simulink model "gtm_aeromodel"  (Simulink 7.2)
settings: Solver=ode45  StartTime=0.0  StopTime=10.0  RelTol=1e-3
undefined symbols (not defined in the file or in its folder): A_BLCG, A_BW, A_CW, A_FSCG, A_FSREF_in, A_SW, A_WLCG, A_WLREF, ALPHA0, bclowb, bclowbx_FMACH, bcmowb, bcmowbx_FHP, bcmowby_FMACH, cda, cdax_FLPDEF, cddr, cddrx_FMACH, cdo, cdox_FLPDEF, cdt1, cdt1x_mach, cdt2, cdt2x_mach, cdto, cdtox_mach, cdwb, cdwbx_FALPHA, cdwby_FMACH, clat, clatfr, clatfrx_FHP, clatfry_FMACH, clatx_mach, clawbfr, clawbfrx_FHP, clawbfry_FMACH, cldefr, cldefrx_FHP, cldefry_FMACH, cldtab, cldtabx_FMACH, clqwb, clqwbfr, clqwbfrx_FHP, clqwbfry_FMACH, clqwbx_mach, cltdd, cltddx_FHP, cltddy_FMACH, clwb, clwbtdd, clwbtddx_FHP, clwbtddy_FMACH, clwbx_FALPHA, clwby_FMACH, clwbzdd, clwbzddx_FHP, clwbzddy_FMACH, clzdd ... (+196)
libraries: model_lib x1
(part 8 of 10)

== system gtm_aeromodel/get aero forces and moments/AERODYNAMICS/Force  Coefficients/LIFT/CLWB/CLWBFLEX ==
  note: tddco2g=fqadot*fcbar/(2*32.174)
  altitude : Inport  OutDataType=sfix(16)  OutScaling=2^0
  Mach : Inport  Port=2  OutDataType=sfix(16)  OutScaling=2^0
  norm acc g's : Inport  Port=3  OutDataType=sfix(16)  OutScaling=2^0
  qdot : Inport  Port=4  OutDataType=sfix(16)  OutScaling=2^0
  Enable : EnablePort
  Fcn1 : Fcn  Expr=1/u
  Product1 : Product  OutDataType=sfix(16)  OutScaling=2^0  SaturateOnIntegerOverflow=on  RndMeth=Zero  InputSameDT=on  OutDataTypeStr=Inherit: Same as first input
  Product2 : Product  Inputs=3  OutDataType=sfix(16)  OutScaling=2^0  SaturateOnIntegerOverflow=on  RndMeth=Zero  InputSameDT=on  OutDataTypeStr=Inherit: Same as first input
  Product3 : Product  OutDataType=sfix(16)  OutScaling=2^0  SaturateOnIntegerOverflow=on  RndMeth=Zero  InputSameDT=on  OutDataTypeStr=Inherit: Same as first input
  Product4 : Product  OutDataType=sfix(16)  OutScaling=2^0  SaturateOnIntegerOverflow=on  RndMeth=Zero  InputSameDT=on  OutDataTypeStr=Inherit: Same as first input
  Sum3 : Sum  OutDataType=sfix(16)  OutScaling=2^0  SaturateOnIntegerOverflow=on  InputSameDT=on  OutDataTypeStr=Inherit: Same as first input
  Wing Chord : Constant  Value=A_CW  OutDataType=sfix(16)  OutScaling=2^0
  Wing Chord1 : Constant  Value=2  OutDataType=sfix(16)  OutScaling=2^0
  Wing Chord2 : Constant  Value=constants.g  OutDataType=sfix(16)  OutScaling=2^0
  clawbfr_ : Subsystem  mask(2-D Table){y=clawbfrx_FHP, z=clawbfry_FMACH, tab=clawbfr}
      mask prompts: y "Y vector:"; z "Z vector:"; tab "Table:"
      mask help: 2-D Table Look Up. Enter monotonic Y and Z vectors and a matrix of 2-D tables. See the help for more info.
      mask Help: The Y and Z vectors must be monotonic.  Y  indexes into the columns of the 2-D table & Z indexes into the rows of the 2-D tables.   The input values are y and z respectively (e.g., top port = y).
      mask Display: plot(-10,-10,110,110,[90,50,10],[90,40,30],[90,50,10],[50,26,20],[90,50,10],[22,13,10])
  clwbtdd : Subsystem  mask(2-D Table){y=clwbtddx_FHP, z=clwbtddy_FMACH, tab=clwbtdd}
      mask prompts: y "Y vector:"; z "Z vector:"; tab "Table:"
      mask help: 2-D Table Look Up. Enter monotonic Y and Z vectors and a matrix of 2-D tables. See the help for more info.
      mask Help: The Y and Z vectors must be monotonic.  Y  indexes into the columns of the 2-D table & Z indexes into the rows of the 2-D tables.   The input values are y and z respectively (e.g., top port = y).
      mask Display: plot(-10,-10,110,110,[90,50,10],[90,40,30],[90,50,10],[50,26,20],[90,50,10],[22,13,10])
  clwbzdd : Subsystem  mask(2-D Table){y=clwbzddx_FHP, z=clwbzddy_FMACH, tab=clwbzdd}
      mask prompts: y "Y vector:"; z "Z vector:"; tab "Table:"
      mask help: 2-D Table Look Up. Enter monotonic Y and Z vectors and a matrix of 2-D tables. See the help for more info.
      mask Help: The Y and Z vectors must be monotonic.  Y  indexes into the columns of the 2-D table & Z indexes into the rows of the 2-D tables.   The input values are y and z respectively (e.g., top port = y).
      mask Display: plot(-10,-10,110,110,[90,50,10],[90,40,30],[90,50,10],[50,26,20],[90,50,10],[22,13,10])
  dclowbflex : Subsystem  mask(2-D Table){y=dclowbflexx_FHP, z=dclowbflexy_FMACH, tab=dclowbflex}
      mask prompts: y "Y vector:"; z "Z vector:"; tab "Table:"
      mask help: 2-D Table Look Up. Enter monotonic Y and Z vectors and a matrix of 2-D tables. See the help for more info.
      mask Help: The Y and Z vectors must be monotonic.  Y  indexes into the columns of the 2-D table & Z indexes into the rows of the 2-D tables.   The input values are y and z respectively (e.g., top port = y).
      mask Display: plot(-10,-10,110,110,[90,50,10],[90,40,30],[90,50,10],[50,26,20],[90,50,10],[22,13,10])
  clawbfr : Outport  OutDataType=sfix(16)  OutScaling=2^0  InitialOutput=0
  cl_flx : Outport  Port=2  OutDataType=sfix(16)  OutScaling=2^0  InitialOutput=0
  fdclowb : Outport  Port=3  OutDataType=sfix(16)  OutScaling=2^0  InitialOutput=0
  wires:
  dclowbflex/1(Interp Value) -> fdclowb/1
  Sum3/1 -> cl_flx/1
  Wing Chord1/1 -> Product4/1
  Fcn1/1 -> Product2/3
  Product3/1 -> Product2/2
  qdot/1 -> Product3/1
  Product4/1 -> Fcn1/1
  Wing Chord2/1 -> Product4/2
  Wing Chord/1 -> Product3/2
  Product2/1 -> Sum3/2
  Product1/1 -> Sum3/1
  norm acc g's/1 -> Product1/2
  clwbtdd/1(Interp Value) -> Product2/1
  clwbzdd/1(Interp Value) -> Product1/1
  clawbfr_/1(Interp Value) -> clawbfr/1
  altitude/1 -> clwbtdd/1(Y), clwbzdd/1(Y), clawbfr_/1(Y), dclowbflex/1(Y)
  Mach/1 -> clwbtdd/2(Z), clwbzdd/2(Z), clawbfr_/2(Z), dclowbflex/2(Z)

== system gtm_aeromodel/get aero forces and moments/AERODYNAMICS/Force  Coefficients/LIFT/CLWB/cl_flap_ ==
  flap : Inport  OutDataType=sfix(16)  OutScaling=2^0
  alpha : Inport  Port=2  OutDataType=sfix(16)  OutScaling=2^0
  qdyn : Inport  Port=3  OutDataType=sfix(16)  OutScaling=2^0
  flex : Inport  Port=4  OutDataType=sfix(16)  OutScaling=2^0
  dsb : Inport  Port=5  OutDataType=sfix(16)  OutScaling=2^0
  Enable : EnablePort
  DSB : Constant  Value=0.0  OutDataType=sfix(16)  OutScaling=2^0
  MACH : Constant  Value=0.178  OutDataType=sfix(16)  OutScaling=2^0
  Product : Product  OutDataType=sfix(16)  OutScaling=2^0  SaturateOnIntegerOverflow=on  RndMeth=Zero  InputSameDT=on  OutDataTypeStr=Inherit: Same as first input
  Sum : Sum  Inputs=+-  OutDataType=sfix(16)  OutScaling=2^0  SaturateOnIntegerOverflow=on  InputSameDT=on  OutDataTypeStr=Inherit: Same as first input
  Sum1 : Sum  Inputs=+--  OutDataType=sfix(16)  OutScaling=2^0  SaturateOnIntegerOverflow=on  InputSameDT=on  OutDataTypeStr=Inherit: Same as first input
  Switch5 : Switch  Threshold=0.5  SaturateOnIntegerOverflow=on  InputSameDT=on
  clwb : Subsystem  mask(2-D Table){y=clwbx_FALPHA, z=clwby_FMACH, tab=clwb}
      mask prompts: y "Y vector:"; z "Z vector:"; tab "Table:"
      mask help: 2-D Table Look Up. Enter monotonic Y and Z vectors and a matrix of 2-D tables. See the help for more info.
      mask Help: The Y and Z vectors must be monotonic.  Y  indexes into the columns of the 2-D table & Z indexes into the rows of the 2-D tables.   The input values are y and z respectively (e.g., top port = y).
      mask Display: plot(-10,-10,110,110,[90,50,10],[90,40,30],[90,50,10],[50,26,20],[90,50,10],[22,13,10])
  clwbdsbdf : Subsystem  mask(1-2-3 Table){@1=clwbdsbdfx_DSB, @2=clwbdsbdfy_FALPHA, @3=clwbdsbdfz_FLPDEF, @4=clwbdsbdf}
      mask prompts: @1 "X vector:"; @2 "Y vector:"; @3 "Z vector:"; @4 "Table:"
      mask help: 3-D Table Look Up. Enter monotonic X, Y and Z vectors and a matrix of 2-D tables. See the help for more info.
      mask init:
      | x=@1;y=@2;z=@3;tab=@4;
      mask Help: The X, Y and Z vectors must be monotonic.   The 3-D table is a horizontal concatenation of  2-D tables.  X  indexes into the columns of the 2-D tables & Y indexes into the rows of the 2-D tables.  Z indexes into the table levels (starting with the 1st 2-D table).   The input values are x, y and z respectively (e.g., top port = x).
      mask Display: plot([0 2 2 0 0],[0 0 2 2 0],[0 2 2.9 0.95 0],[2 2 2.7 2.7 2],[2 2.9 2.9 2 2],[0 0.85 2.7 2 0])
  clwbdsbdf1 : Subsystem  mask(1-2-3 Table){@1=clwbdsbdfx_DSB, @2=clwbdsbdfy_FALPHA, @3=clwbdsbdfz_FLPDEF, @4=clwbdsbdf}
      mask prompts: @1 "X vector:"; @2 "Y vector:"; @3 "Z vector:"; @4 "Table:"
      mask help: 3-D Table Look Up. Enter monotonic X, Y and Z vectors and a matrix of 2-D tables. See the help for more info.
      mask init:
      | x=@1;y=@2;z=@3;tab=@4;
      mask Help: The X, Y and Z vectors must be monotonic.   The 3-D table is a horizontal concatenation of  2-D tables.  X  indexes into the columns of the 2-D tables & Y indexes into the rows of the 2-D tables.  Z indexes into the table levels (starting with the 1st 2-D table).   The input values are x, y and z respectively (e.g., top port = x).
      mask Display: plot([0 2 2 0 0],[0 0 2 2 0],[0 2 2.9 0.95 0],[2 2 2.7 2.7 2],[2 2.9 2.9 2 2],[0 0.85 2.7 2 0])
  const : Constant  Value=1.0  OutDataType=sfix(16)  OutScaling=2^0
  dclwbdffr : Subsystem  mask(2-D Table){y=dclwbdffrx_FQ, z=dclwbdffry_FLPDEF, tab=dclwbdffr}
      mask prompts: y "Y vector:"; z "Z vector:"; tab "Table:"
      mask help: 2-D Table Look Up. Enter monotonic Y and Z vectors and a matrix of 2-D tables. See the help for more info.
      mask Help: The Y and Z vectors must be monotonic.  Y  indexes into the columns of the 2-D table & Z indexes into the rows of the 2-D tables.   The input values are y and z respectively (e.g., top port = y).
      mask Display: plot(-10,-10,110,110,[90,50,10],[90,40,30],[90,50,10],[50,26,20],[90,50,10],[22,13,10])
  dclwbdsbdf : Subsystem  mask(1-2-3 Table){@1=dclwbdsbx_DSB, @2=dclwbdsby_ALPHA, @3=dclwbdsbz_FMACH, @4=dclwbdsb}
      mask prompts: @1 "X vector:"; @2 "Y vector:"; @3 "Z vector:"; @4 "Table:"
      mask help: 3-D Table Look Up. Enter monotonic X, Y and Z vectors and a matrix of 2-D tables. See the help for more info.
      mask init:
      | x=@1;y=@2;z=@3;tab=@4;
      mask Help: The X, Y and Z vectors must be monotonic.   The 3-D table is a horizontal concatenation of  2-D tables.  X  indexes into the columns of the 2-D tables & Y indexes into the rows of the 2-D tables.  Z indexes into the table levels (starting with the 1st 2-D table).   The input values are x, y and z respectively (e.g., top port = x).
      mask Display: plot([0 2 2 0 0],[0 0 2 2 0],[0 2 2.9 0.95 0],[2 2 2.7 2.7 2],[2 2.9 2.9 2 2],[0 0.85 2.7 2 0])
  cl_flap : Outport  OutDataType=sfix(16)  OutScaling=2^0  InitialOutput=0
  dclsbfint : Outport  Port=2  OutDataType=sfix(16)  OutScaling=2^0  InitialOutput=0
  wires:
  Sum1/1 -> dclsbfint/1
  dclwbdffr/1(Interp Value) -> Switch5/1
  clwbdsbdf/1(Interp Value) -> Sum1/2, Sum/1
  clwbdsbdf1/1(Interp Value) -> Sum1/1
  Switch5/1 -> Product/2
  const/1 -> Switch5/3
  flex/1 -> Switch5/2
  qdyn/1 -> dclwbdffr/1(Y)
  Product/1 -> cl_flap/1
  flap/1 -> clwbdsbdf1/3(Z), dclwbdffr/2(Z), clwbdsbdf/3(Z)
  Sum/1 -> Product/1
  alpha/1 -> clwbdsbdf/2(Y), clwbdsbdf1/2(Y), dclwbdsbdf/2(Y), clwb/1(Y)
  DSB/1 -> clwbdsbdf/1(X)
  MACH/1 -> clwb/2(Z), dclwbdsbdf/3(Z)
  dsb/1 -> clwbdsbdf1/1(X), dclwbdsbdf/1(X)
  dclwbdsbdf/1(Interp Value) -> Sum1/3
  clwb/1(Interp Value) -> Sum/2

== system gtm_aeromodel/get aero forces and moments/AERODYNAMICS/Force  Coefficients/LIFT/CLWB/clwb_ ==
  Y : Inport  OutDataType=sfix(16)  OutScaling=2^0
  Z : Inport  Port=2  OutDataType=sfix(16)  OutScaling=2^0
  Mux : Mux  Inputs=2
  S-Function : S-Function  FunctionName=table2v5  Parameters=y,z,tab  EnableBusSupport=off
  Interp Value : Outport  OutDataType=sfix(16)  OutScaling=2^0
  wires:
  Mux/1 -> S-Function/1
  S-Function/1 -> Interp Value/1
  Y/1 -> Mux/1
  Z/1 -> Mux/2

== system gtm_aeromodel/get aero forces and moments/AERODYNAMICS/Force  Coefficients/LIFT/CLWB/clwb_zero ==
  Y : Inport  OutDataType=sfix(16)  OutScaling=2^0
  Z : Inport  Port=2  OutDataType=sfix(16)  OutScaling=2^0
  Mux : Mux  Inputs=2
  S-Function : S-Function  FunctionName=table2v5  Parameters=y,z,tab  EnableBusSupport=off
  Interp Value : Outport  OutDataType=sfix(16)  OutScaling=2^0
  wires:
  Z/1 -> Mux/2
  Y/1 -> Mux/1
  S-Function/1 -> Interp Value/1
  Mux/1 -> S-Function/1

== system gtm_aeromodel/get aero forces and moments/AERODYNAMICS/Force  Coefficients/LIFT/DCLDE/cldefr ==
  altitude : Inport  OutDataType=sfix(16)  OutScaling=2^0
  mach : Inport  Port=2  OutDataType=sfix(16)  OutScaling=2^0
  Enable : EnablePort
  cldefr_ : Subsystem  mask(2-D Table){y=cldefrx_FHP, z=cldefry_FMACH, tab=cldefr}
      mask prompts: y "Y vector:"; z "Z vector:"; tab "Table:"
      mask help: 2-D Table Look Up. Enter monotonic Y and Z vectors and a matrix of 2-D tables. See the help for more info.
      mask Help: The Y and Z vectors must be monotonic.  Y  indexes into the columns of the 2-D table & Z indexes into the rows of the 2-D tables.   The input values are y and z respectively (e.g., top port = y).
      mask Display: plot(-10,-10,110,110,[90,50,10],[90,40,30],[90,50,10],[50,26,20],[90,50,10],[22,13,10])
  cldefr : Outport  OutDataType=sfix(16)  OutScaling=2^0  InitialOutput=0
  wires:
  mach/1 -> cldefr_/2(Z)
  altitude/1 -> cldefr_/1(Y)
  cldefr_/1(Interp Value) -> cldefr/1

== system gtm_aeromodel/get aero forces and moments/AERODYNAMICS/Force  Coefficients/LIFT/DCLDE/dclde_ ==
  X : Inport  OutDataType=sfix(16)  OutScaling=2^0
  Y : Inport  Port=2  OutDataType=sfix(16)  OutScaling=2^0
  Z : Inport  Port=3  OutDataType=sfix(16)  OutScaling=2^0
  Mux : Mux  Inputs=3
  S-Function : S-Function  FunctionName=table3v5  Parameters=x,y,z,tab  EnableBusSupport=off
  Interp Value : Outport  OutDataType=sfix(16)  OutScaling=2^0
  wires:
  Z/1 -> Mux/3
  Y/1 -> Mux/2
  X/1 -> Mux/1
  Mux/1 -> S-Function/1
  S-Function/1 -> Interp Value/1

== system gtm_aeromodel/get aero forces and moments/AERODYNAMICS/Force  Coefficients/LIFT/bclowb/bclowb_ ==
  Z : Inport  OutDataType=sfix(16)  OutScaling=2^0
  S-Function : S-Function  FunctionName=table1v5  Parameters=z,tab  EnableBusSupport=off
  Interp Value : Outport  OutDataType=sfix(16)  OutScaling=2^0
  wires:
  Z/1 -> S-Function/1
  S-Function/1 -> Interp Value/1

== system gtm_aeromodel/get aero forces and moments/AERODYNAMICS/Force  Coefficients/SIDE/CYBWB/CYWBFLEX ==
  altitude : Inport  OutDataType=sfix(16)  OutScaling=2^0
  Mach : Inport  Port=2  OutDataType=sfix(16)  OutScaling=2^0
  Enable : EnablePort
  cybfr_ : Subsystem  mask(2-D Table){y=cybfrx_FHP, z=cybfry_FMACH, tab=cybfr}
      mask prompts: y "Y vector:"; z "Z vector:"; tab "Table:"
      mask help: 2-D Table Look Up. Enter monotonic Y and Z vectors and a matrix of 2-D tables. See the help for more info.
      mask Help: The Y and Z vectors must be monotonic.  Y  indexes into the columns of the 2-D table & Z indexes into the rows of the 2-D tables.   The input values are y and z respectively (e.g., top port = y).
      mask Display: plot(-10,-10,110,110,[90,50,10],[90,40,30],[90,50,10],[50,26,20],[90,50,10],[22,13,10])
  cybfr : Outport  OutDataType=sfix(16)  OutScaling=2^0  InitialOutput=0
  wires:
  cybfr_/1(Interp Value) -> cybfr/1
  altitude/1 -> cybfr_/1(Y)
  Mach/1 -> cybfr_/2(Z)

== system gtm_aeromodel/get aero forces and moments/AERODYNAMICS/Force  Coefficients/SIDE/CYBWB/cy_flap_ ==
  flap : Inport  OutDataType=sfix(16)  OutScaling=2^0
  alpha : Inport  Port=2  OutDataType=sfix(16)  OutScaling=2^0
  Enable : EnablePort
  dcybdf : Subsystem  mask(2-D Table){y=dcybdfx_FLPDEF, z=dcybdfy_FALPHA, tab=dcybdf}
      mask prompts: y "Y vector:"; z "Z vector:"; tab "Table:"
      mask help: 2-D Table Look Up. Enter monotonic Y and Z vectors and a matrix of 2-D tables. See the help for more info.
      mask Help: The Y and Z vectors must be monotonic.  Y  indexes into the columns of the 2-D table & Z indexes into the rows of the 2-D tables.   The input values are y and z respectively (e.g., top port = y).
      mask Display: plot(-10,-10,110,110,[90,50,10],[90,40,30],[90,50,10],[50,26,20],[90,50,10],[22,13,10])
  cy_flap : Outport  OutDataType=sfix(16)  OutScaling=2^0  InitialOutput=0
  wires:
  flap/1 -> dcybdf/1(Y)
  alpha/1 -> dcybdf/2(Z)
  dcybdf/1(Interp Value) -> cy_flap/1

== system gtm_aeromodel/get aero forces and moments/AERODYNAMICS/Force  Coefficients/SIDE/CYBWB/cybwb ==
  Y : Inport  OutDataType=sfix(16)  OutScaling=2^0
  Z : Inport  Port=2  OutDataType=sfix(16)  OutScaling=2^0
  Mux : Mux  Inputs=2
  S-Function : S-Function  FunctionName=table2v5  Parameters=y,z,tab  EnableBusSupport=off
  Interp Value : Outport  OutDataType=sfix(16)  OutScaling=2^0
  wires:
  Mux/1 -> S-Function/1
  S-Function/1 -> Interp Value/1
  Y/1 -> Mux/1
  Z/1 -> Mux/2

== system gtm_aeromodel/get aero forces and moments/AERODYNAMICS/Force  Coefficients/SIDE/CYGEAR/dcyba ==
  Z : Inport  OutDataType=sfix(16)  OutScaling=2^0
  S-Function : S-Function  FunctionName=table1v5  Parameters=z,tab  EnableBusSupport=off
  Interp Value : Outport  OutDataType=sfix(16)  OutScaling=2^0
  wires:
  Z/1 -> S-Function/1
  S-Function/1 -> Interp Value/1

== system gtm_aeromodel/get aero forces and moments/AERODYNAMICS/Force  Coefficients/SIDE/CYGEAR/dcybo ==
  Z : Inport  OutDataType=sfix(16)  OutScaling=2^0
  S-Function : S-Function  FunctionName=table1v5  Parameters=z,tab  EnableBusSupport=off
  Interp Value : Outport  OutDataType=sfix(16)  OutScaling=2^0
  wires:
  Z/1 -> S-Function/1
  S-Function/1 -> Interp Value/1

== system gtm_aeromodel/get aero forces and moments/AERODYNAMICS/Force  Coefficients/SIDE/CYP/CYPFLEX ==
  altitude : Inport  OutDataType=sfix(16)  OutScaling=2^0
  Mach : Inport  Port=2  OutDataType=sfix(16)  OutScaling=2^0
  Enable : EnablePort
  cypfr_ : Subsystem  mask(2-D Table){y=cypfrx_FHP, z=cypfry_FMACH, tab=cypfr}
      mask prompts: y "Y vector:"; z "Z vector:"; tab "Table:"
      mask help: 2-D Table Look Up. Enter monotonic Y and Z vectors and a matrix of 2-D tables. See the help for more info.
      mask Help: The Y and Z vectors must be monotonic.  Y  indexes into the columns of the 2-D table & Z indexes into the rows of the 2-D tables.   The input values are y and z respectively (e.g., top port = y).
      mask Display: plot(-10,-10,110,110,[90,50,10],[90,40,30],[90,50,10],[50,26,20],[90,50,10],[22,13,10])
  cypfr : Outport  OutDataType=sfix(16)  OutScaling=2^0  InitialOutput=0
  wires:
  Mach/1 -> cypfr_/2(Z)
  altitude/1 -> cypfr_/1(Y)
  cypfr_/1(Interp Value) -> cypfr/1

== system gtm_aeromodel/get aero forces and moments/AERODYNAMICS/Force  Coefficients/SIDE/CYP/rcrbvt ==
  Y : Inport  OutDataType=sfix(16)  OutScaling=2^0
  Z : Inport  Port=2  OutDataType=sfix(16)  OutScaling=2^0
  Mux : Mux  Inputs=2
  S-Function : S-Function  FunctionName=table2v5  Parameters=y,z,tab  EnableBusSupport=off
  Interp Value : Outport  OutDataType=sfix(16)  OutScaling=2^0
  wires:
  Mux/1 -> S-Function/1
  S-Function/1 -> Interp Value/1
  Y/1 -> Mux/1
  Z/1 -> Mux/2

== system gtm_aeromodel/get aero forces and moments/AERODYNAMICS/Force  Coefficients/SIDE/CYP/rcybvt ==
  Y : Inport  OutDataType=sfix(16)  OutScaling=2^0
  Z : Inport  Port=2  OutDataType=sfix(16)  OutScaling=2^0
  Mux : Mux  Inputs=2
  S-Function : S-Function  FunctionName=table2v5  Parameters=y,z,tab  EnableBusSupport=off
  Interp Value : Outport  OutDataType=sfix(16)  OutScaling=2^0
  wires:
  Z/1 -> Mux/2
  Y/1 -> Mux/1
  S-Function/1 -> Interp Value/1
  Mux/1 -> S-Function/1

== system gtm_aeromodel/get aero forces and moments/AERODYNAMICS/Force  Coefficients/SIDE/CYP/rcypwb ==
  Y : Inport  OutDataType=sfix(16)  OutScaling=2^0
  Z : Inport  Port=2  OutDataType=sfix(16)  OutScaling=2^0
  Mux : Mux  Inputs=2
  S-Function : S-Function  FunctionName=table2v5  Parameters=y,z,tab  EnableBusSupport=off
  Interp Value : Outport  OutDataType=sfix(16)  OutScaling=2^0
  wires:
  Z/1 -> Mux/2
  Y/1 -> Mux/1
  S-Function/1 -> Interp Value/1
  Mux/1 -> S-Function/1

== system gtm_aeromodel/get aero forces and moments/AERODYNAMICS/Force  Coefficients/SIDE/CYR/CYRFLEX ==
  altitude : Inport  OutDataType=sfix(16)  OutScaling=2^0
  Mach : Inport  Port=2  OutDataType=sfix(16)  OutScaling=2^0
  Enable : EnablePort
  cyrfr_ : Subsystem  mask(2-D Table){y=cyrfrx_FHP, z=cyrfry_FMACH, tab=cyrfr}
      mask prompts: y "Y vector:"; z "Z vector:"; tab "Table:"
      mask help: 2-D Table Look Up. Enter monotonic Y and Z vectors and a matrix of 2-D tables. See the help for more info.
      mask Help: The Y and Z vectors must be monotonic.  Y  indexes into the columns of the 2-D table & Z indexes into the rows of the 2-D tables.   The input values are y and z respectively (e.g., top port = y).
      mask Display: plot(-10,-10,110,110,[90,50,10],[90,40,30],[90,50,10],[50,26,20],[90,50,10],[22,13,10])
  cyrfr : Outport  OutDataType=sfix(16)  OutScaling=2^0  InitialOutput=0
  wires:
  Mach/1 -> cyrfr_/2(Z)
  altitude/1 -> cyrfr_/1(Y)
  cyrfr_/1(Interp Value) -> cyrfr/1

== system gtm_aeromodel/get aero forces and moments/AERODYNAMICS/Force  Coefficients/SIDE/CYR/cnbvt ==
  Y : Inport  OutDataType=sfix(16)  OutScaling=2^0
  Z : Inport  Port=2  OutDataType=sfix(16)  OutScaling=2^0
  Mux : Mux  Inputs=2
  S-Function : S-Function  FunctionName=table2v5  Parameters=y,z,tab  EnableBusSupport=off
  Interp Value : Outport  OutDataType=sfix(16)  OutScaling=2^0
  wires:
  Z/1 -> Mux/2
  Y/1 -> Mux/1
  S-Function/1 -> Interp Value/1
  Mux/1 -> S-Function/1

== system gtm_aeromodel/get aero forces and moments/AERODYNAMICS/Force  Coefficients/SIDE/CYR/cybvt ==
  Y : Inport  OutDataType=sfix(16)  OutScaling=2^0
  Z : Inport  Port=2  OutDataType=sfix(16)  OutScaling=2^0
  Mux : Mux  Inputs=2
  S-Function : S-Function  FunctionName=table2v5  Parameters=y,z,tab  EnableBusSupport=off
  Interp Value : Outport  OutDataType=sfix(16)  OutScaling=2^0
  wires:
  Mux/1 -> S-Function/1
  S-Function/1 -> Interp Value/1
  Y/1 -> Mux/1
  Z/1 -> Mux/2

== system gtm_aeromodel/get aero forces and moments/AERODYNAMICS/Force  Coefficients/SIDE/CYR/rcyrwb ==
  Z : Inport  OutDataType=sfix(16)  OutScaling=2^0
  S-Function : S-Function  FunctionName=table1v5  Parameters=z,tab  EnableBusSupport=off
  Interp Value : Outport  OutDataType=sfix(16)  OutScaling=2^0
  wires:
  S-Function/1 -> Interp Value/1
  Z/1 -> S-Function/1

== system gtm_aeromodel/get aero forces and moments/AERODYNAMICS/Force  Coefficients/SIDE/CYRUD/CYRFLEX ==
  altitude : Inport  OutDataType=sfix(16)  OutScaling=2^0
  Mach : Inport  Port=2  OutDataType=sfix(16)  OutScaling=2^0
  Enable : EnablePort
  cydrfr : Subsystem  mask(2-D Table){y=cydrfrx_FHP, z=cydrfry_FMACH, tab=cydrfr}
      mask prompts: y "Y vector:"; z "Z vector:"; tab "Table:"
      mask help: 2-D Table Look Up. Enter monotonic Y and Z vectors and a matrix of 2-D tables. See the help for more info.
      mask Help: The Y and Z vectors must be monotonic.  Y  indexes into the columns of the 2-D table & Z indexes into the rows of the 2-D tables.   The input values are y and z respectively (e.g., top port = y).
      mask Display: plot(-10,-10,110,110,[90,50,10],[90,40,30],[90,50,10],[50,26,20],[90,50,10],[22,13,10])
  cyrfr : Outport  OutDataType=sfix(16)  OutScaling=2^0  InitialOutput=0
  wires:
  Mach/1 -> cydrfr/2(Z)
  altitude/1 -> cydrfr/1(Y)
  cydrfr/1(Interp Value) -> cyrfr/1

== system gtm_aeromodel/get aero forces and moments/AERODYNAMICS/Force  Coefficients/SIDE/CYRUD/cydr ==
  Z : Inport  OutDataType=sfix(16)  OutScaling=2^0
  S-Function : S-Function  FunctionName=table1v5  Parameters=z,tab  EnableBusSupport=off
  Interp Value : Outport  OutDataType=sfix(16)  OutScaling=2^0
  wires:
  S-Function/1 -> Interp Value/1
  Z/1 -> S-Function/1

== system gtm_aeromodel/get aero forces and moments/AERODYNAMICS/Force  Coefficients/SIDE/CYSPOIL/cy_sp_int ==
  flap : Inport  OutDataType=sfix(16)  OutScaling=2^0
  alpha : Inport  Port=2  OutDataType=sfix(16)  OutScaling=2^0
  dsl : Inport  Port=3  OutDataType=sfix(16)  OutScaling=2^0
  dsb : Inport  Port=4  OutDataType=sfix(16)  OutScaling=2^0
  dsr : Inport  Port=5  OutDataType=sfix(16)  OutScaling=2^0
  Enable : EnablePort
  Sum : Sum  Inputs=+-  OutDataType=sfix(16)  OutScaling=2^0  SaturateOnIntegerOverflow=on  InputSameDT=on  OutDataTypeStr=Inherit: Same as first input
  Sum1 : Sum  Inputs=-+  OutDataType=sfix(16)  OutScaling=2^0  SaturateOnIntegerOverflow=on  InputSameDT=on  OutDataTypeStr=Inherit: Same as first input
  Sum2 : Sum  Inputs=+-  OutDataType=sfix(16)  OutScaling=2^0  SaturateOnIntegerOverflow=on  InputSameDT=on  OutDataTypeStr=Inherit: Same as first input
  dcywbdsldf : Subsystem  mask(1-2-3 Table){@1=dcywbdsldfx_DSL, @2=dcywbdsldfy_FALPHA, @3=dcywbdsldfz_FLPDEF, @4=dcywbdsldf}
      mask prompts: @1 "X vector:"; @2 "Y vector:"; @3 "Z vector:"; @4 "Table:"
      mask help: 3-D Table Look Up. Enter monotonic X, Y and Z vectors and a matrix of 2-D tables. See the help for more info.
      mask init:
      | x=@1;y=@2;z=@3;tab=@4;
      mask Help: The X, Y and Z vectors must be monotonic.   The 3-D table is a horizontal concatenation of  2-D tables.  X  indexes into the columns of the 2-D tables & Y indexes into the rows of the 2-D tables.  Z indexes into the table levels (starting with the 1st 2-D table).   The input values are x, y and z respectively (e.g., top port = x).
      mask Display: plot([0 2 2 0 0],[0 0 2 2 0],[0 2 2.9 0.95 0],[2 2 2.7 2.7 2],[2 2.9 2.9 2 2],[0 0.85 2.7 2 0])
  dcywbdsldf1 : Subsystem  mask(1-2-3 Table){@1=dcywbdsldfx_DSL, @2=dcywbdsldfy_FALPHA, @3=dcywbdsldfz_FLPDEF, @4=dcywbdsldf}
      mask prompts: @1 "X vector:"; @2 "Y vector:"; @3 "Z vector:"; @4 "Table:"
      mask help: 3-D Table Look Up. Enter monotonic X, Y and Z vectors and a matrix of 2-D tables. See the help for more info.
      mask init:
      | x=@1;y=@2;z=@3;tab=@4;
      mask Help: The X, Y and Z vectors must be monotonic.   The 3-D table is a horizontal concatenation of  2-D tables.  X  indexes into the columns of the 2-D tables & Y indexes into the rows of the 2-D tables.  Z indexes into the table levels (starting with the 1st 2-D table).   The input values are x, y and z respectively (e.g., top port = x).
      mask Display: plot([0 2 2 0 0],[0 0 2 2 0],[0 2 2.9 0.95 0],[2 2 2.7 2.7 2],[2 2.9 2.9 2 2],[0 0.85 2.7 2 0])
  dcywbdsldf_ : Subsystem  mask(1-2-3 Table){@1=dcywbdsldfx_DSL, @2=dcywbdsldfy_FALPHA, @3=dcywbdsldfz_FLPDEF, @4=dcywbdsldf}
      mask prompts: @1 "X vector:"; @2 "Y vector:"; @3 "Z vector:"; @4 "Table:"
      mask help: 3-D Table Look Up. Enter monotonic X, Y and Z vectors and a matrix of 2-D tables. See the help for more info.
      mask init:
      | x=@1;y=@2;z=@3;tab=@4;
      mask Help: The X, Y and Z vectors must be monotonic.   The 3-D table is a horizontal concatenation of  2-D tables.  X  indexes into the columns of the 2-D tables & Y indexes into the rows of the 2-D tables.  Z indexes into the table levels (starting with the 1st 2-D table).   The input values are x, y and z respectively (e.g., top port = x).
      mask Display: plot([0 2 2 0 0],[0 0 2 2 0],[0 2 2.9 0.95 0],[2 2 2.7 2.7 2],[2 2.9 2.9 2 2],[0 0.85 2.7 2 0])
  cy_spfl_int : Outport  OutDataType=sfix(16)  OutScaling=2^0  InitialOutput=0
  wires:
  dsl/1 -> dcywbdsldf/1(X)
  alpha/1 -> dcywbdsldf_/2(Y), dcywbdsldf1/2(Y), dcywbdsldf/2(Y)
  dcywbdsldf/1(Interp Value) -> Sum/1
  flap/1 -> dcywbdsldf/3(Z), dcywbdsldf_/3(Z), dcywbdsldf1/3(Z)
  dcywbdsldf1/1(Interp Value) -> Sum1/2
  dcywbdsldf_/1(Interp Value) -> Sum/2, Sum1/1
  Sum/1 -> Sum2/1
  Sum1/1 -> Sum2/2
  Sum2/1 -> cy_spfl_int/1
  dsb/1 -> dcywbdsldf_/1(X)
  dsr/1 -> dcywbdsldf1/1(X)

== system gtm_aeromodel/get aero forces and moments/AERODYNAMICS/Force  Coefficients/SIDE/CYSPOIL/dcywbdsl ==
  X : Inport  OutDataType=sfix(16)  OutScaling=2^0
  Y : Inport  Port=2  OutDataType=sfix(16)  OutScaling=2^0
  Z : Inport  Port=3  OutDataType=sfix(16)  OutScaling=2^0
  Mux : Mux  Inputs=3
  S-Function : S-Function  FunctionName=table3v5  Parameters=x,y,z,tab  EnableBusSupport=off
  Interp Value : Outport  OutDataType=sfix(16)  OutScaling=2^0
  wires:
  S-Function/1 -> Interp Value/1
  Mux/1 -> S-Function/1
  X/1 -> Mux/1
  Y/1 -> Mux/2
  Z/1 -> Mux/3

== system gtm_aeromodel/get aero forces and moments/AERODYNAMICS/Force  Coefficients/SIDE/CYSPOIL/dcywbdsl1 ==
  X : Inport  OutDataType=sfix(16)  OutScaling=2^0
  Y : Inport  Port=2  OutDataType=sfix(16)  OutScaling=2^0
  Z : Inport  Port=3  OutDataType=sfix(16)  OutScaling=2^0
  Mux : Mux  Inputs=3
  S-Function : S-Function  FunctionName=table3v5  Parameters=x,y,z,tab  EnableBusSupport=off
  Interp Value : Outport  OutDataType=sfix(16)  OutScaling=2^0
  wires:
  Z/1 -> Mux/3
  Y/1 -> Mux/2
  X/1 -> Mux/1
  Mux/1 -> S-Function/1
  S-Function/1 -> Interp Value/1

== system gtm_aeromodel/get aero forces and moments/AERODYNAMICS/Force  Coefficients/SIDE/CYSPOIL/dcywbdsl2 ==
  X : Inport  OutDataType=sfix(16)  OutScaling=2^0
  Y : Inport  Port=2  OutDataType=sfix(16)  OutScaling=2^0
  Z : Inport  Port=3  OutDataType=sfix(16)  OutScaling=2^0
  Mux : Mux  Inputs=3
  S-Function : S-Function  FunctionName=table3v5  Parameters=x,y,z,tab  EnableBusSupport=off
  Interp Value : Outport  OutDataType=sfix(16)  OutScaling=2^0
  wires:
  Z/1 -> Mux/3
  Y/1 -> Mux/2
  X/1 -> Mux/1
  Mux/1 -> S-Function/1
  S-Function/1 -> Interp Value/1

== system gtm_aeromodel/get aero forces and moments/AERODYNAMICS/Force  Coefficients/SIDE/CYSPOIL/dcywbdsl3 ==
  X : Inport  OutDataType=sfix(16)  OutScaling=2^0
  Y : Inport  Port=2  OutDataType=sfix(16)  OutScaling=2^0
  Z : Inport  Port=3  OutDataType=sfix(16)  OutScaling=2^0
  Mux : Mux  Inputs=3
  S-Function : S-Function  FunctionName=table3v5  Parameters=x,y,z,tab  EnableBusSupport=off
  Interp Value : Outport  OutDataType=sfix(16)  OutScaling=2^0
  wires:
  Z/1 -> Mux/3
  Y/1 -> Mux/2
  X/1 -> Mux/1
  Mux/1 -> S-Function/1
  S-Function/1 -> Interp Value/1

== system gtm_aeromodel/get aero forces and moments/AERODYNAMICS/Force  Coefficients/SIDE/CYSPOIL/dcywbdsl4 ==
  X : Inport  OutDataType=sfix(16)  OutScaling=2^0
  Y : Inport  Port=2  OutDataType=sfix(16)  OutScaling=2^0
  Z : Inport  Port=3  OutDataType=sfix(16)  OutScaling=2^0
  Mux : Mux  Inputs=3
  S-Function : S-Function  FunctionName=table3v5  Parameters=x,y,z,tab  EnableBusSupport=off
  Interp Value : Outport  OutDataType=sfix(16)  OutScaling=2^0
  wires:
  Z/1 -> Mux/3
  Y/1 -> Mux/2
  X/1 -> Mux/1
  Mux/1 -> S-Function/1
  S-Function/1 -> Interp Value/1

== system gtm_aeromodel/get aero forces and moments/AERODYNAMICS/Force  Coefficients/SIDE/CYSPOIL/dcywbdsl5 ==
  X : Inport  OutDataType=sfix(16)  OutScaling=2^0
  Y : Inport  Port=2  OutDataType=sfix(16)  OutScaling=2^0
  Z : Inport  Port=3  OutDataType=sfix(16)  OutScaling=2^0
  Mux : Mux  Inputs=3
  S-Function : S-Function  FunctionName=table3v5  Parameters=x,y,z,tab  EnableBusSupport=off
  Interp Value : Outport  OutDataType=sfix(16)  OutScaling=2^0
  wires:
  Z/1 -> Mux/3
  Y/1 -> Mux/2
  X/1 -> Mux/1
  Mux/1 -> S-Function/1
  S-Function/1 -> Interp Value/1

== system gtm_aeromodel/get aero forces and moments/AERODYNAMICS/Force  Coefficients/SIDE/TAIL/cybht ==
  Y : Inport  OutDataType=sfix(16)  OutScaling=2^0
  Z : Inport  Port=2  OutDataType=sfix(16)  OutScaling=2^0
  Mux : Mux  Inputs=2
  S-Function : S-Function  FunctionName=table2v5  Parameters=y,z,tab  EnableBusSupport=off
  Interp Value : Outport  OutDataType=sfix(16)  OutScaling=2^0
  wires:
  Z/1 -> Mux/2
  Y/1 -> Mux/1
  S-Function/1 -> Interp Value/1
  Mux/1 -> S-Function/1

== system gtm_aeromodel/get aero forces and moments/AERODYNAMICS/Force  Coefficients/SIDE/TAIL/cybvt ==
  Y : Inport  OutDataType=sfix(16)  OutScaling=2^0
  Z : Inport  Port=2  OutDataType=sfix(16)  OutScaling=2^0
  Mux : Mux  Inputs=2
  S-Function : S-Function  FunctionName=table2v5  Parameters=y,z,tab  EnableBusSupport=off
  Interp Value : Outport  OutDataType=sfix(16)  OutScaling=2^0
  wires:
  Mux/1 -> S-Function/1
  S-Function/1 -> Interp Value/1
  Y/1 -> Mux/1
  Z/1 -> Mux/2

== system gtm_aeromodel/get aero forces and moments/AERODYNAMICS/Moment Coefficients/PITCH/BCMOWB/cmatfr ==
  Y : Inport  OutDataType=sfix(16)  OutScaling=2^0
  Z : Inport  Port=2  OutDataType=sfix(16)  OutScaling=2^0
  Mux : Mux  Inputs=2
  S-Function : S-Function  FunctionName=table2v5  Parameters=y,z,tab  EnableBusSupport=off
  Interp Value : Outport  OutDataType=sfix(16)  OutScaling=2^0
  wires:
  Z/1 -> Mux/2
  Y/1 -> Mux/1
  S-Function/1 -> Interp Value/1
  Mux/1 -> S-Function/1

== system gtm_aeromodel/get aero forces and moments/AERODYNAMICS/Moment Coefficients/PITCH/CMQWB/cmqwb_ ==
  Z : Inport  OutDataType=sfix(16)  OutScaling=2^0
  S-Function : S-Function  FunctionName=table1v5  Parameters=z,tab  EnableBusSupport=off
  Interp Value : Outport  OutDataType=sfix(16)  OutScaling=2^0
  wires:
  Z/1 -> S-Function/1
  S-Function/1 -> Interp Value/1

== system gtm_aeromodel/get aero forces and moments/AERODYNAMICS/Moment Coefficients/PITCH/CMQWB/cmqwbfr ==
  altitude : Inport  OutDataType=sfix(16)  OutScaling=2^0
  mach1 : Inport  Port=2  OutDataType=sfix(16)  OutScaling=2^0
  Enable : EnablePort
  cmqwbfr_ : Subsystem  mask(2-D Table){y=cmqwbfrx_FHP, z=cmqwbfry_FMACH, tab=cmqwbfr}
      mask prompts: y "Y vector:"; z "Z vector:"; tab "Table:"
      mask help: 2-D Table Look Up. Enter monotonic Y and Z vectors and a matrix of 2-D tables. See the help for more info.
      mask Help: The Y and Z vectors must be monotonic.  Y  indexes into the columns of the 2-D table & Z indexes into the rows of the 2-D tables.   The input values are y and z respectively (e.g., top port = y).
      mask Display: plot(-10,-10,110,110,[90,50,10],[90,40,30],[90,50,10],[50,26,20],[90,50,10],[22,13,10])
  cmqwbfr : Outport  OutDataType=sfix(16)  OutScaling=2^0  InitialOutput=0
  wires:
  cmqwbfr_/1(Interp Value) -> cmqwbfr/1
  mach1/1 -> cmqwbfr_/2(Z)
  altitude/1 -> cmqwbfr_/1(Y)

== system gtm_aeromodel/get aero forces and moments/AERODYNAMICS/Moment Coefficients/PITCH/CMSPOIL/cm_sp_int ==
  flap : Inport  OutDataType=sfix(16)  OutScaling=2^0
  alpha : Inport  Port=2  OutDataType=sfix(16)  OutScaling=2^0
  dsl : Inport  Port=3  OutDataType=sfix(16)  OutScaling=2^0
  dsb : Inport  Port=4  OutDataType=sfix(16)  OutScaling=2^0
  dsr : Inport  Port=5  OutDataType=sfix(16)  OutScaling=2^0
  Enable : EnablePort
  Sum : Sum  Inputs=+-  OutDataType=sfix(16)  OutScaling=2^0  SaturateOnIntegerOverflow=on  InputSameDT=on  OutDataTypeStr=Inherit: Same as first input
  Sum1 : Sum  Inputs=-+  OutDataType=sfix(16)  OutScaling=2^0  SaturateOnIntegerOverflow=on  InputSameDT=on  OutDataTypeStr=Inherit: Same as first input
  Sum2 : Sum  OutDataType=sfix(16)  OutScaling=2^0  SaturateOnIntegerOverflow=on  InputSameDT=on  OutDataTypeStr=Inherit: Same as first input
  dcmwbdsbp : Subsystem  mask(1-2-3 Table){@1=dcmwbdsldfx_DSL, @2=dcmwbdsldfy_FALPHA, @3=dcmwbdsldfz_FLPDEF, @4=dcmwbdsldf}
      mask prompts: @1 "X vector:"; @2 "Y vector:"; @3 "Z vector:"; @4 "Table:"
      mask help: 3-D Table Look Up. Enter monotonic X, Y and Z vectors and a matrix of 2-D tables. See the help for more info.
      mask init:
      | x=@1;y=@2;z=@3;tab=@4;
      mask Help: The X, Y and Z vectors must be monotonic.   The 3-D table is a horizontal concatenation of  2-D tables.  X  indexes into the columns of the 2-D tables & Y indexes into the rows of the 2-D tables.  Z indexes into the table levels (starting with the 1st 2-D table).   The input values are x, y and z respectively (e.g., top port = x).
      mask Display: plot([0 2 2 0 0],[0 0 2 2 0],[0 2 2.9 0.95 0],[2 2 2.7 2.7 2],[2 2.9 2.9 2 2],[0 0.85 2.7 2 0])
  dcmwbdsldf : Subsystem  mask(1-2-3 Table){@1=dcmwbdsldfx_DSL, @2=dcmwbdsldfy_FALPHA, @3=dcmwbdsldfz_FLPDEF, @4=dcmwbdsldf}
      mask prompts: @1 "X vector:"; @2 "Y vector:"; @3 "Z vector:"; @4 "Table:"
      mask help: 3-D Table Look Up. Enter monotonic X, Y and Z vectors and a matrix of 2-D tables. See the help for more info.
      mask init:
      | x=@1;y=@2;z=@3;tab=@4;
      mask Help: The X, Y and Z vectors must be monotonic.   The 3-D table is a horizontal concatenation of  2-D tables.  X  indexes into the columns of the 2-D tables & Y indexes into the rows of the 2-D tables.  Z indexes into the table levels (starting with the 1st 2-D table).   The input values are x, y and z respectively (e.g., top port = x).
      mask Display: plot([0 2 2 0 0],[0 0 2 2 0],[0 2 2.9 0.95 0],[2 2 2.7 2.7 2],[2 2.9 2.9 2 2],[0 0.85 2.7 2 0])
  dcmwbdsldf1 : Subsystem  mask(1-2-3 Table){@1=dcmwbdsldfx_DSL, @2=dcmwbdsldfy_FALPHA, @3=dcmwbdsldfz_FLPDEF, @4=dcmwbdsldf}
      mask prompts: @1 "X vector:"; @2 "Y vector:"; @3 "Z vector:"; @4 "Table:"
      mask help: 3-D Table Look Up. Enter monotonic X, Y and Z vectors and a matrix of 2-D tables. See the help for more info.
      mask init:
      | x=@1;y=@2;z=@3;tab=@4;
      mask Help: The X, Y and Z vectors must be monotonic.   The 3-D table is a horizontal concatenation of  2-D tables.  X  indexes into the columns of the 2-D tables & Y indexes into the rows of the 2-D tables.  Z indexes into the table levels (starting with the 1st 2-D table).   The input values are x, y and z respectively (e.g., top port = x).
      mask Display: plot([0 2 2 0 0],[0 0 2 2 0],[0 2 2.9 0.95 0],[2 2 2.7 2.7 2],[2 2.9 2.9 2 2],[0 0.85 2.7 2 0])
  cm_sp_int : Outport  OutDataType=sfix(16)  OutScaling=2^0  InitialOutput=0
  wires:
  Sum1/1 -> Sum2/2
  Sum/1 -> Sum2/1
  Sum2/1 -> cm_sp_int/1
  dcmwbdsbp/1(Interp Value) -> Sum1/1, Sum/2
  dcmwbdsldf1/1(Interp Value) -> Sum1/2
  flap/1 -> dcmwbdsldf/3(Z), dcmwbdsbp/3(Z), dcmwbdsldf1/3(Z)
  dcmwbdsldf/1(Interp Value) -> Sum/1
  alpha/1 -> dcmwbdsldf/2(Y), dcmwbdsbp/2(Y), dcmwbdsldf1/2(Y)
  dsl/1 -> dcmwbdsldf/1(X)
  dsb/1 -> dcmwbdsbp/1(X)
  dsr/1 -> dcmwbdsldf1/1(X)

== system gtm_aeromodel/get aero forces and moments/AERODYNAMICS/Moment Coefficients/PITCH/CMSPOIL/dcmdsbfr ==
  flex : Inport  OutDataType=sfix(16)  OutScaling=2^0
  altitude : Inport  Port=2  OutDataType=sfix(16)  OutScaling=2^0
  mach : Inport  Port=3  OutDataType=sfix(16)  OutScaling=2^0
  Switch7 : Switch  Threshold=0.5  SaturateOnIntegerOverflow=on  InputSameDT=on
  dcmdsbfr_ : Subsystem  mask(2-D Table){y=dcmdsbfrx_FHP, z=dcmdsbfry_FMACH, tab=dcmdsbfr}
      mask prompts: y "Y vector:"; z "Z vector:"; tab "Table:"
      mask help: 2-D Table Look Up. Enter monotonic Y and Z vectors and a matrix of 2-D tables. See the help for more info.
      mask Help: The Y and Z vectors must be monotonic.  Y  indexes into the columns of the 2-D table & Z indexes into the rows of the 2-D tables.   The input values are y and z respectively (e.g., top port = y).
      mask Display: plot(-10,-10,110,110,[90,50,10],[90,40,30],[90,50,10],[50,26,20],[90,50,10],[22,13,10])
  one : Constant  OutDataType=sfix(16)  OutScaling=2^0
  dcmdsbfr : Outport  OutDataType=sfix(16)  OutScaling=2^0  InitialOutput=0
  wires:
  Switch7/1 -> dcmdsbfr/1
  dcmdsbfr_/1(Interp Value) -> Switch7/1
  one/1 -> Switch7/3
  flex/1 -> Switch7/2
  mach/1 -> dcmdsbfr_/2(Z)
  altitude/1 -> dcmdsbfr_/1(Y)

== system gtm_aeromodel/get aero forces and moments/AERODYNAMICS/Moment Coefficients/PITCH/CMSPOIL/dcmwbdsb ==
  X : Inport  OutDataType=sfix(16)  OutScaling=2^0
  Y : Inport  Port=2  OutDataType=sfix(16)  OutScaling=2^0
  Z : Inport  Port=3  OutDataType=sfix(16)  OutScaling=2^0
  Mux : Mux  Inputs=3
  S-Function : S-Function  FunctionName=table3v5  Parameters=x,y,z,tab  EnableBusSupport=off
  Interp Value : Outport  OutDataType=sfix(16)  OutScaling=2^0
  wires:
  Z/1 -> Mux/3
  Y/1 -> Mux/2
  X/1 -> Mux/1
  Mux/1 -> S-Function/1
  S-Function/1 -> Interp Value/1

== system gtm_aeromodel/get aero forces and moments/AERODYNAMICS/Moment Coefficients/PITCH/CMSPOIL/dcmwbdsb_ ==
  X : Inport  OutDataType=sfix(16)  OutScaling=2^0
  Y : Inport  Port=2  OutDataType=sfix(16)  OutScaling=2^0
  Z : Inport  Port=3  OutDataType=sfix(16)  OutScaling=2^0
  Mux : Mux  Inputs=3
  S-Function : S-Function  FunctionName=table3v5  Parameters=x,y,z,tab  EnableBusSupport=off
  Interp Value : Outport  OutDataType=sfix(16)  OutScaling=2^0
  wires:
  S-Function/1 -> Interp Value/1
  Mux/1 -> S-Function/1
  X/1 -> Mux/1
  Y/1 -> Mux/2
  Z/1 -> Mux/3

== system gtm_aeromodel/get aero forces and moments/AERODYNAMICS/Moment Coefficients/PITCH/CMSPOIL/dcmwbdsl ==
  X : Inport  OutDataType=sfix(16)  OutScaling=2^0
  Y : Inport  Port=2  OutDataType=sfix(16)  OutScaling=2^0
  Z : Inport  Port=3  OutDataType=sfix(16)  OutScaling=2^0
  Mux : Mux  Inputs=3
  S-Function : S-Function  FunctionName=table3v5  Parameters=x,y,z,tab  EnableBusSupport=off
  Interp Value : Outport  OutDataType=sfix(16)  OutScaling=2^0
  wires:
  Z/1 -> Mux/3
  Y/1 -> Mux/2
  X/1 -> Mux/1
  Mux/1 -> S-Function/1
  S-Function/1 -> Interp Value/1

== system gtm_aeromodel/get aero forces and moments/AERODYNAMICS/Moment Coefficients/PITCH/CMSPOIL/dcmwbdsl1 ==
  X : Inport  OutDataType=sfix(16)  OutScaling=2^0
  Y : Inport  Port=2  OutDataType=sfix(16)  OutScaling=2^0
  Z : Inport  Port=3  OutDataType=sfix(16)  OutScaling=2^0
  Mux : Mux  Inputs=3
  S-Function : S-Function  FunctionName=table3v5  Parameters=x,y,z,tab  EnableBusSupport=off
  Interp Value : Outport  OutDataType=sfix(16)  OutScaling=2^0
  wires:
  S-Function/1 -> Interp Value/1
  Mux/1 -> S-Function/1
  X/1 -> Mux/1
  Y/1 -> Mux/2
  Z/1 -> Mux/3

== system gtm_aeromodel/get aero forces and moments/AERODYNAMICS/Moment Coefficients/PITCH/CMSPOIL/dcmwbdsl_ ==
  X : Inport  OutDataType=sfix(16)  OutScaling=2^0
  Y : Inport  Port=2  OutDataType=sfix(16)  OutScaling=2^0
  Z : Inport  Port=3  OutDataType=sfix(16)  OutScaling=2^0
  Mux : Mux  Inputs=3
  S-Function : S-Function  FunctionName=table3v5  Parameters=x,y,z,tab  EnableBusSupport=off
  Interp Value : Outport  OutDataType=sfix(16)  OutScaling=2^0
  wires:
  S-Function/1 -> Interp Value/1
  Mux/1 -> S-Function/1
  X/1 -> Mux/1
  Y/1 -> Mux/2
  Z/1 -> Mux/3

== system gtm_aeromodel/get aero forces and moments/AERODYNAMICS/Moment Coefficients/PITCH/CMSPOIL/dcmwbdsl_1 ==
  X : Inport  OutDataType=sfix(16)  OutScaling=2^0
  Y : Inport  Port=2  OutDataType=sfix(16)  OutScaling=2^0
  Z : Inport  Port=3  OutDataType=sfix(16)  OutScaling=2^0
  Mux : Mux  Inputs=3
  S-Function : S-Function  FunctionName=table3v5  Parameters=x,y,z,tab  EnableBusSupport=off
  Interp Value : Outport  OutDataType=sfix(16)  OutScaling=2^0
  wires:
  Z/1 -> Mux/3
  Y/1 -> Mux/2
  X/1 -> Mux/1
  Mux/1 -> S-Function/1
  S-Function/1 -> Interp Value/1

== system gtm_aeromodel/get aero forces and moments/AERODYNAMICS/Moment Coefficients/PITCH/CMSPOIL/dcmwbdsl_2 ==
  X : Inport  OutDataType=sfix(16)  OutScaling=2^0
  Y : Inport  Port=2  OutDataType=sfix(16)  OutScaling=2^0
  Z : Inport  Port=3  OutDataType=sfix(16)  OutScaling=2^0
  Mux : Mux  Inputs=3
  S-Function : S-Function  FunctionName=table3v5  Parameters=x,y,z,tab  EnableBusSupport=off
  Interp Value : Outport  OutDataType=sfix(16)  OutScaling=2^0
  wires:
  S-Function/1 -> Interp Value/1
  Mux/1 -> S-Function/1
  X/1 -> Mux/1
  Y/1 -> Mux/2
  Z/1 -> Mux/3

== system gtm_aeromodel/get aero forces and moments/AERODYNAMICS/Moment Coefficients/PITCH/CMSPOIL/dcmwbdsl_3 ==
  X : Inport  OutDataType=sfix(16)  OutScaling=2^0
  Y : Inport  Port=2  OutDataType=sfix(16)  OutScaling=2^0
  Z : Inport  Port=3  OutDataType=sfix(16)  OutScaling=2^0
  Mux : Mux  Inputs=3
  S-Function : S-Function  FunctionName=table3v5  Parameters=x,y,z,tab  EnableBusSupport=off
  Interp Value : Outport  OutDataType=sfix(16)  OutScaling=2^0
  wires:
  Z/1 -> Mux/3
  Y/1 -> Mux/2
  X/1 -> Mux/1
  Mux/1 -> S-Function/1
  S-Function/1 -> Interp Value/1

== system gtm_aeromodel/get aero forces and moments/AERODYNAMICS/Moment Coefficients/PITCH/CMT/CMAT ==
  Z : Inport  OutDataType=sfix(16)  OutScaling=2^0
  S-Function : S-Function  FunctionName=table1v5  Parameters=z,tab  EnableBusSupport=off
  Interp Value : Outport  OutDataType=sfix(16)  OutScaling=2^0
  wires:
  Z/1 -> S-Function/1
  S-Function/1 -> Interp Value/1

== system gtm_aeromodel/get aero forces and moments/AERODYNAMICS/Moment Coefficients/PITCH/CMT/cltailfx ==
  note: tddco2g=fqadot*fcbar/(2*32.174)
  altitude : Inport  OutDataType=sfix(16)  OutScaling=2^0
  Mach : Inport  Port=2  OutDataType=sfix(16)  OutScaling=2^0
  norm acc g's : Inport  Port=3  OutDataType=sfix(16)  OutScaling=2^0
  qdot : Inport  Port=4  OutDataType=sfix(16)  OutScaling=2^0
  Enable : EnablePort
  Fcn1 : Fcn  Expr=1/u
  Product1 : Product  OutDataType=sfix(16)  OutScaling=2^0  SaturateOnIntegerOverflow=on  RndMeth=Zero  InputSameDT=on  OutDataTypeStr=Inherit: Same as first input
  Product2 : Product  Inputs=3  OutDataType=sfix(16)  OutScaling=2^0  SaturateOnIntegerOverflow=on  RndMeth=Zero  InputSameDT=on  OutDataTypeStr=Inherit: Same as first input
  Product3 : Product  OutDataType=sfix(16)  OutScaling=2^0  SaturateOnIntegerOverflow=on  RndMeth=Zero  InputSameDT=on  OutDataTypeStr=Inherit: Same as first input
  Product4 : Product  OutDataType=sfix(16)  OutScaling=2^0  SaturateOnIntegerOverflow=on  RndMeth=Zero  InputSameDT=on  OutDataTypeStr=Inherit: Same as first input
  Sum2 : Sum  OutDataType=sfix(16)  OutScaling=2^0  SaturateOnIntegerOverflow=on  InputSameDT=on  OutDataTypeStr=Inherit: Same as first input
  Wing Chord : Constant  Value=A_CW  OutDataType=sfix(16)  OutScaling=2^0
  Wing Chord1 : Constant  Value=2  OutDataType=sfix(16)  OutScaling=2^0
  Wing Chord2 : Constant  Value=constants.g  OutDataType=sfix(16)  OutScaling=2^0
  cmatfr_ : Subsystem  mask(2-D Table){y=cmatfrx_FHP, z=cmatfry_FMACH, tab=cmatfr}
      mask prompts: y "Y vector:"; z "Z vector:"; tab "Table:"
      mask help: 2-D Table Look Up. Enter monotonic Y and Z vectors and a matrix of 2-D tables. See the help for more info.
      mask Help: The Y and Z vectors must be monotonic.  Y  indexes into the columns of the 2-D table & Z indexes into the rows of the 2-D tables.   The input values are y and z respectively (e.g., top port = y).
      mask Display: plot(-10,-10,110,110,[90,50,10],[90,40,30],[90,50,10],[50,26,20],[90,50,10],[22,13,10])
  cmtdd : Subsystem  mask(2-D Table){y=cmtddx_FHP, z=cmtddy_FMACH, tab=cmtdd}
      mask prompts: y "Y vector:"; z "Z vector:"; tab "Table:"
      mask help: 2-D Table Look Up. Enter monotonic Y and Z vectors and a matrix of 2-D tables. See the help for more info.
      mask Help: The Y and Z vectors must be monotonic.  Y  indexes into the columns of the 2-D table & Z indexes into the rows of the 2-D tables.   The input values are y and z respectively (e.g., top port = y).
      mask Display: plot(-10,-10,110,110,[90,50,10],[90,40,30],[90,50,10],[50,26,20],[90,50,10],[22,13,10])
  cmzdd : Subsystem  mask(2-D Table){y=cmzddx_FHP, z=cmzddy_FMACH, tab=cmzdd}
      mask prompts: y "Y vector:"; z "Z vector:"; tab "Table:"
      mask help: 2-D Table Look Up. Enter monotonic Y and Z vectors and a matrix of 2-D tables. See the help for more info.
      mask Help: The Y and Z vectors must be monotonic.  Y  indexes into the columns of the 2-D table & Z indexes into the rows of the 2-D tables.   The input values are y and z respectively (e.g., top port = y).
      mask Display: plot(-10,-10,110,110,[90,50,10],[90,40,30],[90,50,10],[50,26,20],[90,50,10],[22,13,10])
  cmatfr : Outport  OutDataType=sfix(16)  OutScaling=2^0  InitialOutput=0
  cmtflx : Outport  Port=2  OutDataType=sfix(16)  OutScaling=2^0  InitialOutput=0
  wires:
  Product2/1 -> Sum2/2
  Product1/1 -> Sum2/1
  Mach/1 -> cmzdd/2(Z), cmtdd/2(Z), cmatfr_/2(Z)
  cmtdd/1(Interp Value) -> Product2/1
  cmzdd/1(Interp Value) -> Product1/1
  norm acc g's/1 -> Product1/2
  Sum2/1 -> cmtflx/1
  Wing Chord/1 -> Product3/2
  Wing Chord2/1 -> Product4/2
  Product4/1 -> Fcn1/1
  Product3/1 -> Product2/2
  Wing Chord1/1 -> Product4/1
  Fcn1/1 -> Product2/3
  qdot/1 -> Product3/1
  altitude/1 -> cmtdd/1(Y), cmzdd/1(Y), cmatfr_/1(Y)
  cmatfr_/1(Interp Value) -> cmatfr/1

== system gtm_aeromodel/get aero forces and moments/AERODYNAMICS/Moment Coefficients/PITCH/CMTAB/cmdetabfr ==
  alt : Inport  OutDataType=sfix(16)  OutScaling=2^0
  mach : Inport  Port=2  OutDataType=sfix(16)  OutScaling=2^0
  Enable : EnablePort
  cmdetabfr_ : Subsystem  mask(2-D Table){y=cmdetabfrx_altitude, z=cmdetabfry_FMACH, tab=cmdetabfr}
      mask prompts: y "Y vector:"; z "Z vector:"; tab "Table:"
      mask help: 2-D Table Look Up. Enter monotonic Y and Z vectors and a matrix of 2-D tables. See the help for more info.
      mask Help: The Y and Z vectors must be monotonic.  Y  indexes into the columns of the 2-D table & Z indexes into the rows of the 2-D tables.   The input values are y and z respectively (e.g., top port = y).
      mask Display: plot(-10,-10,110,110,[90,50,10],[90,40,30],[90,50,10],[50,26,20],[90,50,10],[22,13,10])
  Out1 : Outport  OutDataType=sfix(16)  OutScaling=2^0
  wires:
  alt/1 -> cmdetabfr_/1(Y)
  mach/1 -> cmdetabfr_/2(Z)
  cmdetabfr_/1(Interp Value) -> Out1/1

== system gtm_aeromodel/get aero forces and moments/AERODYNAMICS/Moment Coefficients/PITCH/CMTAB/cmdtab_ ==
  Z : Inport  OutDataType=sfix(16)  OutScaling=2^0
  S-Function : S-Function  FunctionName=table1v5  Parameters=z,tab  EnableBusSupport=off
  Interp Value : Outport  OutDataType=sfix(16)  OutScaling=2^0
  wires:
  Z/1 -> S-Function/1
  S-Function/1 -> Interp Value/1
